simulink model "test_grid1"  (R2018b)
settings: Solver=ode45  StartTime=0.0  StopTime=10.0  RelTol=1e-3  EnableMultiTasking=on
libraries: powerlib x27
settings Model: Creator=VRIKOS  LastModifiedBy=VRIKOS
settings DataIOCC: LimitDataPoints=on  SaveFormat=Array  SignalLoggingSaveFormat=ModelDataLogs
settings OptimizationCC: ExpressionDepthLimit=2147483647  LifeSpan=inf
settings DebuggingCC: UnderspecifiedInitializationDetection=Classic  MergeDetectMultiDrivingBlocksExec=none  SolverPrmCheckMsg=warning  FcnCallInpInsideContextMsg=warning  StateNameClashWarn=warning  SFUnexpectedBacktrackingDiag=warning  SFNoUnconditionalDefaultTransitionDiag=warning  SFExecutionAtInitializationDiag=none
settings HardwareCC: ProdBitPerPointer=32  ProdBitPerSizeT=32  ProdBitPerPtrDiffT=32  ProdLargestAtomicFloat=None  ProdIntDivRoundTo=Undefined  ProdEndianess=Unspecified  ProdWordSize=32  ProdHWDeviceType=32-bit Generic
settings ModelReferenceCC: PropagateSignalLabelsOutOfModel=off
settings SFSimCC: SimUseLocalCustomCode=off
settings RTWCC: RTWUseLocalCustomCode=off
settings CodeAppCC: StateflowObjectComments=on
settings GRTTargetCC: TargetLangStandard=C89/C90 (ANSI)  GeneratePreprocessorConditionals=Disable all  CombineOutputUpdateFcns=off  GRTInterface=on
settings ConfigComp: CovMetricSettings=dw  CovHtmlReporting=on  CovSaveCumulativeToWorkspaceVar=on  CovSaveSingleToWorkspaceVar=on  CovExternalEMLEnable=off
settings SimscapeCC: SimscapeNormalizeSystem=off

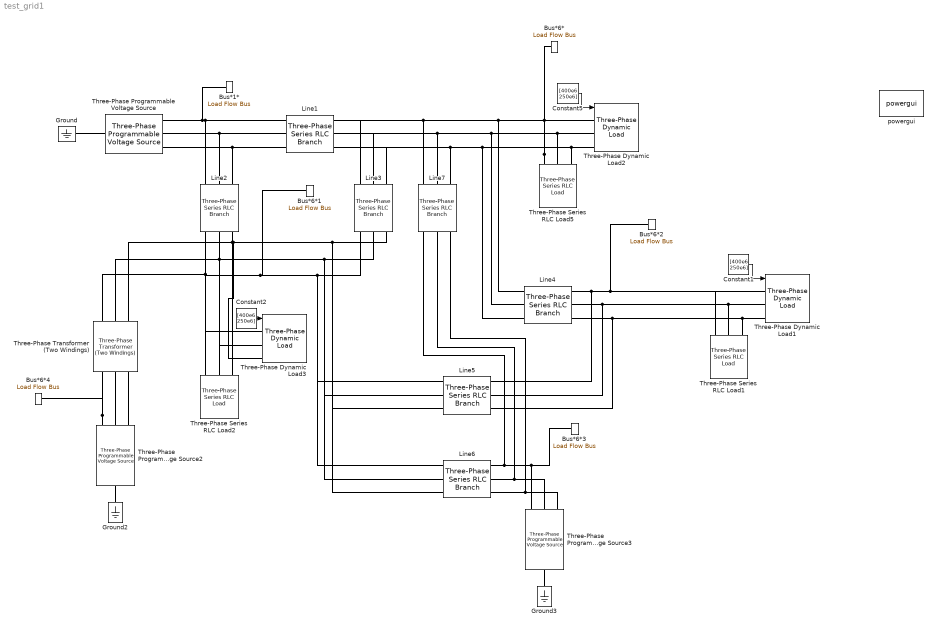
== system test_grid1 ==
  Bus*1* : powerlib/Measurements/Load Flow Bus  LConnTagsString=a  Phases=single  Connectors=on one side  ID=Bus*1*  Vbase=150e3  Vref=1.05  Vangle=0  VLF=1  VLFb=1  VLFc=1  angleLF=0  angleLFb=0  angleLFc=0
      settings: SourceProductName=Simscape Electrical
  Bus*6* : powerlib/Measurements/Load Flow Bus  LConnTagsString=a  Phases=single  Connectors=on one side  ID=Bus*2*  Vbase=150e3  Vref=1  Vangle=0  VLF=1  VLFb=1  VLFc=1  angleLF=0  angleLFb=0  angleLFc=0
      settings: SourceProductName=Simscape Electrical
  Bus*6*1 : powerlib/Measurements/Load Flow Bus  LConnTagsString=a  Phases=single  Connectors=on one side  ID=Bus*3*  Vbase=150e3  Vref=1.04  Vangle=0  VLF=1  VLFb=1  VLFc=1  angleLF=0  angleLFb=0  angleLFc=0
      settings: SourceProductName=Simscape Electrical
  Bus*6*2 : powerlib/Measurements/Load Flow Bus  LConnTagsString=a  Phases=single  Connectors=on one side  ID=Bus*4*  Vbase=150e3  Vref=1  Vangle=0  VLF=1  VLFb=1  VLFc=1  angleLF=0  angleLFb=0  angleLFc=0
      settings: SourceProductName=Simscape Electrical
  Bus*6*3 : powerlib/Measurements/Load Flow Bus  LConnTagsString=a  Phases=single  Connectors=on one side  ID=Bus*5*  Vbase=150e3  Vref=1.04  Vangle=0  VLF=1  VLFb=1  VLFc=1  angleLF=0  angleLFb=0  angleLFc=0
      settings: SourceProductName=Simscape Electrical
  Bus*6*4 : powerlib/Measurements/Load Flow Bus  LConnTagsString=a  Phases=single  Connectors=on one side  ID=Bus*6*  Vbase=150e3  Vref=0.133  Vangle=0  VLF=1  VLFb=1  VLFc=1  angleLF=0  angleLFb=0  angleLFc=0
      settings: SourceProductName=Simscape Electrical
  Constant1 : Constant  Value=[400e6 250e6]
  Constant2 : Constant  Value=[400e6 250e6]
  Constant5 : Constant  Value=[400e6 250e6]
  Ground : powerlib/Elements/Ground  LConnTagsString=a
      settings: SourceProductName=Simscape Electrical
  Ground2 : powerlib/Elements/Ground  LConnTagsString=a
      settings: SourceProductName=Simscape Electrical
  Ground3 : powerlib/Elements/Ground  LConnTagsString=a
      settings: SourceProductName=Simscape Electrical
  Line{1,4..6} (4 alike) : powerlib/Elements/Three-Phase Series RLC Branch  LConnTagsString=A|B|C  RConnTagsString=A|B|C  BranchType=RL  Resistance=4.5  Inductance=9/(2*pi*50)  Capacitance=1e-6  Measurements=None
      settings: SourceProductName=Simscape Electrical
  Line2 : powerlib/Elements/Three-Phase Series RLC Branch  LConnTagsString=A|B|C  RConnTagsString=A|B|C  BranchType=RL  Resistance=2.25  Inductance=6.75/(2*pi*50)  Capacitance=1e-6  Measurements=None
      settings: SourceProductName=Simscape Electrical
  Line3 : powerlib/Elements/Three-Phase Series RLC Branch  LConnTagsString=A|B|C  RConnTagsString=A|B|C  BranchType=RL  Resistance=2.8125  Inductance=5.625/(2*pi*50)  Capacitance=1e-6  Measurements=None
      settings: SourceProductName=Simscape Electrical
  Line7 : powerlib/Elements/Three-Phase Series RLC Branch  LConnTagsString=A|B|C  RConnTagsString=A|B|C  BranchType=RL  Resistance=2.25  Inductance=6.75/(2*pi*50)  Capacitance=1e-6  Measurements=None
      settings: SourceProductName=Simscape Electrical
  Three-Phase Dynamic Load1 : powerlib/Elements/Three-Phase Dynamic Load  NominalVoltage=[ 150e3 50 ]  ActiveReactivePowers=[350e6 250e6]  PositiveSequence=[1 0]  ExternalControl=on  NpNq=[1.3 2]  TimeConstants="[0  0  0  0]"  MinimumVoltage=0.7  Tfilter=1e-4  LoadFlowParameters=[4 100 0 0 100]
      settings: SourceProductName=Simscape Electrical  SourceProductBaseCode=PS
  Three-Phase Dynamic Load2 : powerlib/Elements/Three-Phase Dynamic Load  NominalVoltage=[ 150e3 50 ]  ActiveReactivePowers=[400e6 250e6]  PositiveSequence=[1 0]  ExternalControl=on  NpNq=[1.3 2]  TimeConstants="[0  0  0  0]"  MinimumVoltage=0.7  Tfilter=1e-4  LoadFlowParameters=[4 100 0 0 100]
      settings: SourceProductName=Simscape Electrical  SourceProductBaseCode=PS
  Three-Phase Dynamic Load3 : powerlib/Elements/Three-Phase Dynamic Load  NominalVoltage=[ 150e3 50 ]  ActiveReactivePowers=[100e6 100e6]  PositiveSequence=[1 0]  ExternalControl=on  NpNq=[1.3 2]  TimeConstants="[0  0  0  0]"  MinimumVoltage=0.7  Tfilter=1e-4  LoadFlowParameters=[4 100 0 0 100]
      settings: SourceProductName=Simscape Electrical  SourceProductBaseCode=PS
  Three-Phase Programmable Voltage Source : powerlib/Electrical Sources/Three-Phase Programmable Voltage Source  PositiveSequence=[(150e3)*1.05 0 50]  VariationEntity=None  VariationType=Step  VariationTypeAlt=Step  VariationStep=0.5  VariationRate=10  VariationMagnitude=0.3  VariationFrequency=2  VariationTiming=[1 2]  VariationPhaseA=off  Amplitudes=[1 0.8 1.2 1.0]  TimeValues=[0 0.1 0.15 0.2]  HarmonicGeneration=off  HarmonicA=[3 0.2 -25 0]  HarmonicB=[2 0.15 35 2]  Timing="[0.05  3]"  BusType=swing  Pref=0  Qref=0  Qmin=-inf  Qmax=inf
      settings: SourceProductName=Simscape Electrical
  Three-Phase Programmable Voltage Source2 : powerlib/Electrical Sources/Three-Phase Programmable Voltage Source  PositiveSequence=[(20e3)*1. 0 50]  VariationEntity=None  VariationType=Step  VariationTypeAlt=Step  VariationStep=0.5  VariationRate=10  VariationMagnitude=0.3  VariationFrequency=2  VariationTiming=[1 2]  VariationPhaseA=off  Amplitudes=[1 0.8 1.2 1.0]  TimeValues=[0 0.1 0.15 0.2]  HarmonicGeneration=off  HarmonicA=[3 0.2 -25 0]  HarmonicB=[2 0.15 35 2]  Timing="[0.05  3]"  BusType=PV  Pref=200e6  Qref=0  Qmin=-inf  Qmax=inf
      settings: SourceProductName=Simscape Electrical
  Three-Phase Programmable Voltage Source3 : powerlib/Electrical Sources/Three-Phase Programmable Voltage Source  PositiveSequence=[(150e3)*1.04 0 50]  VariationEntity=None  VariationType=Step  VariationTypeAlt=Step  VariationStep=0.5  VariationRate=10  VariationMagnitude=0.3  VariationFrequency=2  VariationTiming=[1 2]  VariationPhaseA=off  Amplitudes=[1 0.8 1.2 1.0]  TimeValues=[0 0.1 0.15 0.2]  HarmonicGeneration=off  HarmonicA=[3 0.2 -25 0]  HarmonicB=[2 0.15 35 2]  Timing="[0.05  3]"  BusType=PV  Pref=200e6  Qref=0  Qmin=-inf  Qmax=inf
      settings: SourceProductName=Simscape Electrical
  Three-Phase Series RLC Load1 : powerlib/Elements/Three-Phase Series RLC Load  LConnTagsString=A|B|C  Configuration=Y (grounded)  NominalVoltage=150e3  Vabc=[1e3 1e3 1e3]  Vabcp=[1e3 1e3 1e3]  NominalFrequency=50  UnbalancedPower=off  ActivePower=100  InductivePower=0  CapacitivePower=0  Pabc=[10e3 9e3 11e3]  QLabc=[100 90 110]  QCabc=[100 90 110]  Pabcp=[10e3 9e3 11e3]  QLabcp=[100 90 110]  QCabcp=[100 90 110]  Measurements=None  LoadType=constant PQ
      settings: SourceProductName=Simscape Electrical
  Three-Phase Series RLC Load2 : powerlib/Elements/Three-Phase Series RLC Load  LConnTagsString=A|B|C  Configuration=Y (grounded)  NominalVoltage=150e3  Vabc=[1e3 1e3 1e3]  Vabcp=[1e3 1e3 1e3]  NominalFrequency=50  UnbalancedPower=off  ActivePower=100  InductivePower=0  CapacitivePower=0  Pabc=[10e3 9e3 11e3]  QLabc=[100 90 110]  QCabc=[100 90 110]  Pabcp=[10e3 9e3 11e3]  QLabcp=[100 90 110]  QCabcp=[100 90 110]  Measurements=None  LoadType=constant PQ
      settings: SourceProductName=Simscape Electrical
  Three-Phase Series RLC Load5 : powerlib/Elements/Three-Phase Series RLC Load  LConnTagsString=A|B|C  Configuration=Y (grounded)  NominalVoltage=150e3  Vabc=[1e3 1e3 1e3]  Vabcp=[1e3 1e3 1e3]  NominalFrequency=50  UnbalancedPower=off  ActivePower=100  InductivePower=0  CapacitivePower=0  Pabc=[10e3 9e3 11e3]  QLabc=[100 90 110]  QCabc=[100 90 110]  Pabcp=[10e3 9e3 11e3]  QLabcp=[100 90 110]  QCabcp=[100 90 110]  Measurements=None  LoadType=constant PQ
      settings: SourceProductName=Simscape Electrical
  Three-Phase Transformer (Two Windings) : powerlib/Elements/Three-Phase Transformer (Two Windings)  Winding1Connection=Yg  Winding2Connection=Yg  CoreType=Three single-phase transformers  SetSaturation=off  Hysteresis=off  DataFile='hysteresis'  SetInitialFlux=off  Measurements=None  UNITS=SI  NominalPower=[ 25e6 , 50 ]  Winding1=[20e3 0.052822 1.42196/(2*pi*50)]  Winding2=[150e3 0 0]  Rm=1.7288e+07  Lm=145.96*1000  L0=0.025465  Saturation=[0 0;680.27 99297;2.8345e+05 1.2578e+05]  InitialFluxes=[66196 -66196 57921]  MoreParameters=off  BreakLoop=off  DataType=on  TransfoNumber=1
      settings: SourceProductName=Simscape Electrical
  powergui : powerlib/powergui  Priority=1  SimulationMode=Phasor  SampleTime=50e-6  frequency=50  Iterations=15  frequencyindice=50  Pbase=100e6  ErrMax=1e-08  UnitsV=kV  UnitsW=MW  buscounter=8  FunctionMessages=off  echomessages=off  EnableUseOfTLC=off  CurrentSourceSwitches=off  DisableSnubberDevices=off  DisableRonSwitches=off  DisableVfSwitches=off  DisplayEquations=off  SolverType=Tustin/Backward Euler (TBE)  Interpol=off  ExternalGateDelay=off  methode=off  Ts=100  x0status=blocks  SPID=off  SwTol=0  HookPort=off  RestoreLinks=warning  ResistiveCurrentMeasurement=off  Frange=[0:2:500]  Ylog=off  Xlog=on  ShowGrid=off  save=off  variable=ZData  structure=0  ZoomFFT=off  StartTime=0.0  cycles=1  DisplayStyle=1  fundamental=60  FreqAxis=off  MaxFrequency=1000  frequencyindicesteady=1  RmsSteady=1  display=off
      settings: SourceProductName=Simscape Electrical
  wires:
  Constant5/1 -> Three-Phase Dynamic Load2/1
  Constant1/1 -> Three-Phase Dynamic Load1/1
  Constant2/1 -> Three-Phase Dynamic Load3/1
  connections:
  Ground/LConn1 -- Three-Phase Programmable Voltage Source/LConn1
  Three-Phase Series RLC Load5/LConn1 -- Line7/LConn1 -- Line3/LConn1 -- Line1/LConn1 -- Line4/RConn1 -- Three-Phase Dynamic Load2/LConn1 -- Bus*6*/LConn1
  Three-Phase Dynamic Load2/LConn2 -- Line7/LConn2 -- Line3/LConn2 -- Line1/LConn2 -- Line4/RConn2 -- Three-Phase Series RLC Load5/LConn2
  Three-Phase Series RLC Load5/LConn3 -- Line7/LConn3 -- Line3/LConn3 -- Line1/LConn3 -- Line4/RConn3 -- Three-Phase Dynamic Load2/LConn3
  Line1/RConn1 -- Bus*1*/LConn1 -- Three-Phase Programmable Voltage Source/RConn1 -- Line2/LConn1
  Line1/RConn2 -- Line2/LConn2 -- Three-Phase Programmable Voltage Source/RConn2
  Line1/RConn3 -- Line2/LConn3 -- Three-Phase Programmable Voltage Source/RConn3
  Bus*6*1/LConn1 -- Three-Phase Transformer (Two Windings)/RConn1 -- Three-Phase Dynamic Load3/LConn1 -- Three-Phase Series RLC Load2/LConn1 -- Line2/RConn1 -- Line6/RConn1 -- Line5/RConn1 -- Line3/RConn1
  Line2/RConn2 -- Three-Phase Transformer (Two Windings)/RConn2 -- Three-Phase Series RLC Load2/LConn2 -- Three-Phase Dynamic Load3/LConn2 -- Line6/RConn2 -- Line5/RConn2 -- Line3/RConn2
  Line2/RConn3 -- Three-Phase Transformer (Two Windings)/RConn3 -- Three-Phase Series RLC Load2/LConn3 -- Three-Phase Dynamic Load3/LConn3 -- Line6/RConn3 -- Line5/RConn3 -- Line3/RConn3
  Bus*6*2/LConn1 -- Three-Phase Series RLC Load1/LConn1 -- Three-Phase Dynamic Load1/LConn1 -- Line5/LConn1 -- Line4/LConn1
  Line4/LConn2 -- Line5/LConn2 -- Three-Phase Series RLC Load1/LConn2 -- Three-Phase Dynamic Load1/LConn2
  Line4/LConn3 -- Line5/LConn3 -- Three-Phase Series RLC Load1/LConn3 -- Three-Phase Dynamic Load1/LConn3
  Line6/LConn1 -- Line7/RConn1 -- Bus*6*3/LConn1 -- Three-Phase Programmable Voltage Source3/RConn1
  Three-Phase Programmable Voltage Source3/RConn2 -- Line6/LConn2 -- Line7/RConn2
  Three-Phase Programmable Voltage Source3/RConn3 -- Line7/RConn3 -- Line6/LConn3
  Ground3/LConn1 -- Three-Phase Programmable Voltage Source3/LConn1
  Ground2/LConn1 -- Three-Phase Programmable Voltage Source2/LConn1
  Three-Phase Programmable Voltage Source2/RConn1 -- Three-Phase Transformer (Two Windings)/LConn1 -- Bus*6*4/LConn1
  Three-Phase Transformer (Two Windings)/LConn2 -- Three-Phase Programmable Voltage Source2/RConn2
  Three-Phase Transformer (Two Windings)/LConn3 -- Three-Phase Programmable Voltage Source2/RConn3
